simulink model "Current_control"  (R2018a)
settings: Solver=VariableStepAuto  StartTime=0.0  StopTime=10.0  RelTol=1e-3
settings Model: Creator=shami  LastModifiedBy=shami

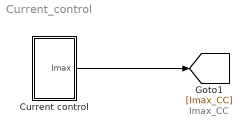
== system Current_control ==
  note: Imax_CC
  Current control : Subsystem
  wires:
  Current control/1(Imax) -> [Imax_CC]

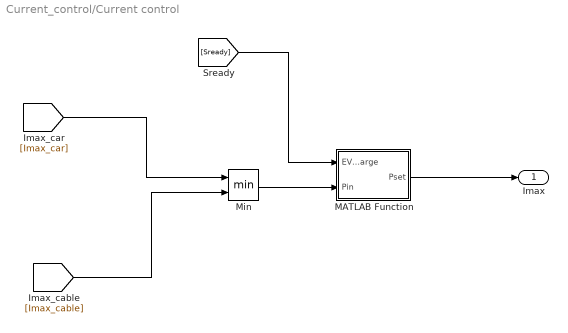
== system Current_control/Current control ==
  MATLAB Function : MATLAB Function  TreatAsAtomicUnit=on
  Min : MinMax  Inputs=2
  Imax : Outport
  wires:
  MATLAB Function/1(Pset) -> Imax/1
  Min/1 -> MATLAB Function/2(Pin)
  [Imax_cable] -> Min/2
  [Sready] -> MATLAB Function/1(EV_charge)
  [Imax_car] -> Min/1

== matlab function Current_control/Current control/MATLAB Function ==
  data: EV_charge input; Pset output; Pin input
function Pset = fcn(EV_charge, Pin)
if EV_charge == 1
    Pset = Pin;
else
    Pset = 0;
end
